simulink model "switch_test"  (Simulink 8.4)
settings: Solver=FixedStepDiscrete  StartTime=0.0  StopTime=10.0  FixedStep=1.0  RelTol=1e-3
settings Model: Creator=arnaud  LastModifiedBy=arnaud
settings DataIOCC: SaveFormat=Structure

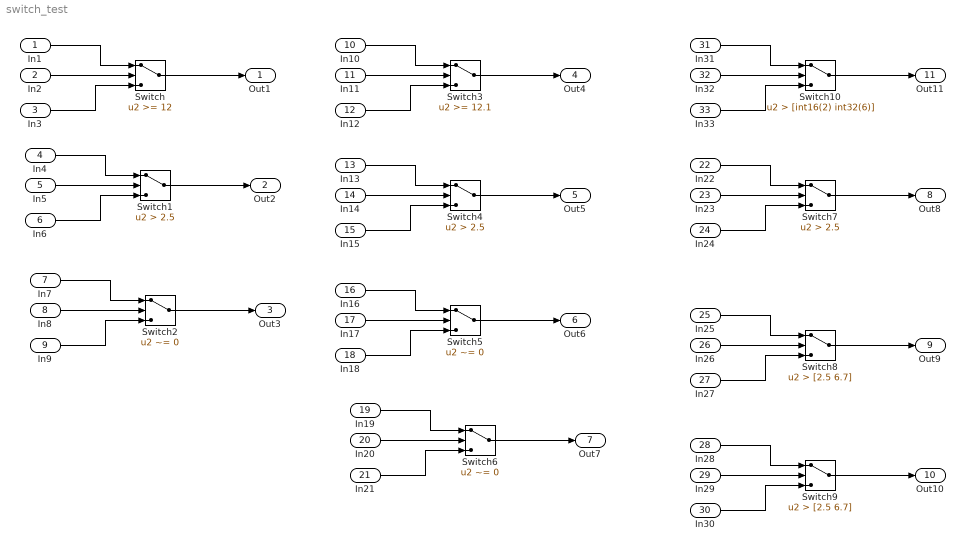
== system switch_test ==
  In1 : Inport
  In2 : Inport  Port=2  OutDataTypeStr=int8
  In3 : Inport  Port=3
  In4 : Inport  Port=4  PortDimensions=[2]
  In5 : Inport  Port=5  OutDataTypeStr=boolean
  In6 : Inport  Port=6  PortDimensions=[2]
  In7 : Inport  Port=7  PortDimensions=[2 3]
  In8 : Inport  Port=8  OutDataTypeStr=boolean
  In9 : Inport  Port=9  PortDimensions=[2 3]
  In10 : Inport  Port=10
  In11 : Inport  Port=11  OutDataTypeStr=double
  In12 : Inport  Port=12
  In13 : Inport  Port=13  PortDimensions=[2]
  In14 : Inport  Port=14  OutDataTypeStr=double
  In15 : Inport  Port=15  PortDimensions=[2]
  In16 : Inport  Port=16  PortDimensions=[2 3]
  In17 : Inport  Port=17  OutDataTypeStr=int16
  In18 : Inport  Port=18  PortDimensions=[2 3]
  In19 : Inport  Port=19  PortDimensions=[2 3]
  In20 : Inport  Port=20  OutDataTypeStr=double
  In21 : Inport  Port=21  PortDimensions=[2 3]
  In22 : Inport  Port=22  PortDimensions=[2]
  In23 : Inport  Port=23  OutDataTypeStr=double  PortDimensions=2
  In24 : Inport  Port=24  PortDimensions=[2]
  In25 : Inport  Port=25  PortDimensions=[2]
  In26 : Inport  Port=26  OutDataTypeStr=double  PortDimensions=2
  In27 : Inport  Port=27  PortDimensions=[2]
  In28 : Inport  Port=28  PortDimensions=[2]
  In29 : Inport  Port=29  OutDataTypeStr=boolean  PortDimensions=2
  In30 : Inport  Port=30  PortDimensions=[2]
  In31 : Inport  Port=31  PortDimensions=[2]
  In32 : Inport  Port=32  OutDataTypeStr=boolean  PortDimensions=2
  In33 : Inport  Port=33  PortDimensions=[2]
  Switch : Switch  Threshold=12
  Switch1 : Switch  Criteria=u2 > Threshold  Threshold=2.5
  Switch10 : Switch  Criteria=u2 > Threshold  Threshold=[int16(2) int32(6)]
  Switch2 : Switch  Criteria=u2 ~= 0
  Switch3 : Switch  Threshold=12.1
  Switch4 : Switch  Criteria=u2 > Threshold  Threshold=2.5
  Switch5 : Switch  Criteria=u2 ~= 0
  Switch6 : Switch  Criteria=u2 ~= 0
  Switch7 : Switch  Criteria=u2 > Threshold  Threshold=2.5
  Switch8 : Switch  Criteria=u2 > Threshold  Threshold=[2.5 6.7]
  Switch9 : Switch  Criteria=u2 > Threshold  Threshold=[2.5 6.7]
  Out1 : Outport
  Out2 : Outport  Port=2
  Out3 : Outport  Port=3
  Out4 : Outport  Port=4
  Out5 : Outport  Port=5
  Out6 : Outport  Port=6
  Out7 : Outport  Port=7
  Out8 : Outport  Port=8
  Out9 : Outport  Port=9
  Out10 : Outport  Port=10
  Out11 : Outport  Port=11
  wires:
  In1/1 -> Switch/1
  In2/1 -> Switch/2
  In3/1 -> Switch/3
  Switch/1 -> Out1/1
  In4/1 -> Switch1/1
  In5/1 -> Switch1/2
  In6/1 -> Switch1/3
  Switch1/1 -> Out2/1
  In7/1 -> Switch2/1
  In8/1 -> Switch2/2
  In9/1 -> Switch2/3
  Switch2/1 -> Out3/1
  In10/1 -> Switch3/1
  In11/1 -> Switch3/2
  In12/1 -> Switch3/3
  Switch3/1 -> Out4/1
  In13/1 -> Switch4/1
  In14/1 -> Switch4/2
  In15/1 -> Switch4/3
  Switch4/1 -> Out5/1
  In16/1 -> Switch5/1
  In17/1 -> Switch5/2
  In18/1 -> Switch5/3
  Switch5/1 -> Out6/1
  In19/1 -> Switch6/1
  In20/1 -> Switch6/2
  In21/1 -> Switch6/3
  Switch6/1 -> Out7/1
  In22/1 -> Switch7/1
  In23/1 -> Switch7/2
  In24/1 -> Switch7/3
  Switch7/1 -> Out8/1
  In25/1 -> Switch8/1
  In26/1 -> Switch8/2
  In27/1 -> Switch8/3
  Switch8/1 -> Out9/1
  In28/1 -> Switch9/1
  In29/1 -> Switch9/2
  In30/1 -> Switch9/3
  Switch9/1 -> Out10/1
  In31/1 -> Switch10/1
  In32/1 -> Switch10/2
  In33/1 -> Switch10/3
  Switch10/1 -> Out11/1
